simulink model "PFE_2Lignes_RNA (2)"  (R2024a)
settings: Solver=ode4  StartTime=0.0  StopTime=0.18  RelTol=1e-3
libraries: neural x202, spsRMSLib x12, spsThreePhasePISectionLineLib x4, spsThreePhaseFaultLib x2, spsThreePhaseVIMeasurementLib x2, spsThreePhaseSourceLib x2, spspowerguiLib x1
(part 6 of 10)

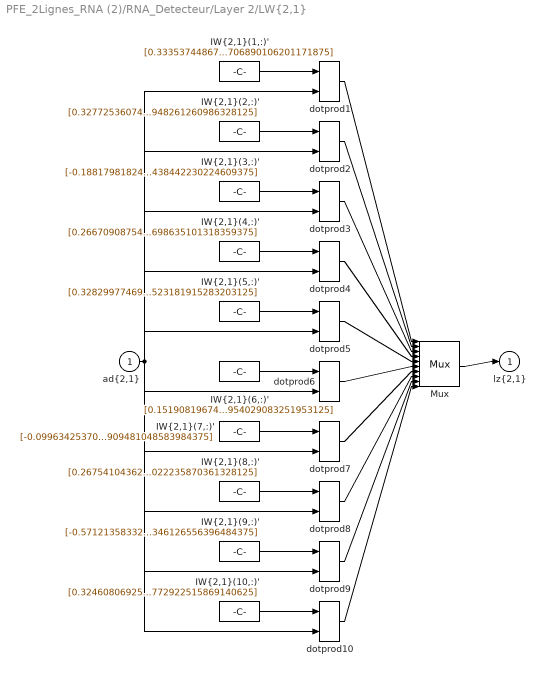
== system PFE_2Lignes_RNA (2)/RNA_Detecteur/Layer 2/LW{2,1} ==
  "ad{2,1}" : Inport  PortDimensions=20
      mask Display: e = 0.06;c1 = [120 230 180]/255;c2 = ([120 230 180]+0)/(256+128);c3 = ([120 230 180]+128)/(256+128);patch([0 1 1 0],[0 0 1 1],c1);patch([0 1 1 1-e 1-e 0+e],[0 0 1 1-e 0+e 0+e],c2);patch([0 0 1 1-e 0+e 0+e],[0 1 1 1-e 1-e 0+e],c3);plot([0 1 1 0 0],[0 0 1 1 0]);
  "IW{2,1}(1,:)'" : Constant  Value=[0.333537448675894021565824232311570085585117340087890625;0.30756652099067094408013645079336129128932952880859375;0.64409548539656069632286516934982500970363616943359375;-0.3189649752100456314707344063208438456058502197265625;0.52701815370737514765409059691592119634151458740234375;0.8021791800394260096851439811871387064456939697265625;-0.2047151820317727466402857317007146775722503662109375;0.6402572386032165940861204944667406380176544189453125;-0.38583498400512439285847676728735677897930145263671875;0.336875538549642195018662960137589834630489349365234375;-0.39560723879220571763681846277904696762561798095703125;-0.2296917297907994370831374908448196947574615478515625;-0.086281908860037670461196057658526115119457244873046875;0.75323236356745859598760262088035233318805694580078125;0.2248015108226981972894265027207438834011554718017578125;-0.50941598680687005806788647532812319695949554443359375;-0.27835551742671615915725169543293304741382598876953125;0.2520155164091217869781758054159581661224365234375;-0.04902099493881727221289423823691322468221187591552734375;-0.40351438380255089111159350068191997706890106201171875]
      mask Display: e = 0.06;c1 = [120 150 230]/255;c2 = ([120 150 230]+0)/383;c3 = ([120 150 230]+128)/383;patch([0 1 1 0],[0 0 1 1],c1);patch([0 1 1 1-e 1-e 0+e],[0 0 1 1-e 0+e 0+e],c2);patch([0 0 1 1-e 0+e 0+e],[0 1 1 1-e 1-e 0+e],c3);plot([0 1 1 0 0],[0 0 1 1 0]);disp('weights');
  "IW{2,1}(10,:)'" : Constant  Value=[0.324608069254977815720764056095504201948642730712890625;-0.2253504424986294274457776509734685532748699188232421875;-0.095126980031401797699430744614801369607448577880859375;0.51391657056152695304263033904135227203369140625;-0.421058213936082392780946292987209744751453399658203125;-0.51267445575505299348861854014103300869464874267578125;-0.443177419805164785060469512245617806911468505859375;0.54168123706777671078071989541058428585529327392578125;0.24154099575073162409211136036901734769344329833984375;0.5612737432708019280624966995674185454845428466796875;-0.1550336204058526401450279763594153337180614471435546875;-0.366469949178925336052969896627473644912242889404296875;-0.0643645953356131172995446831919252872467041015625;-0.295342281285747798591501123155467212200164794921875;0.1845011685122251166024653912245412357151508331298828125;-0.2238883823583790733113829674039152450859546661376953125;0.2272050380486201615060082303898525424301624298095703125;-0.056797317874076568011698640248141600750386714935302734375;-0.3580455383989205042638559461920522153377532958984375;-0.368046203087687262556215728181996382772922515869140625]
      mask Display: e = 0.06;c1 = [120 150 230]/255;c2 = ([120 150 230]+0)/383;c3 = ([120 150 230]+128)/383;patch([0 1 1 0],[0 0 1 1],c1);patch([0 1 1 1-e 1-e 0+e],[0 0 1 1-e 0+e 0+e],c2);patch([0 0 1 1-e 0+e 0+e],[0 1 1 1-e 1-e 0+e],c3);plot([0 1 1 0 0],[0 0 1 1 0]);disp('weights');
  "IW{2,1}(2,:)'" : Constant  Value=[0.3277253607455403727755083309602923691272735595703125;-0.303727259487383050018394214930594898760318756103515625;-0.1794389215878750831745236382630537264049053192138671875;0.1333451232571218891820308272144757211208343505859375;0.317561858062614110753685281451907940208911895751953125;-0.282004928282138578321536215298692695796489715576171875;0.50880406770246455749884262331761419773101806640625;0.451055460360104965022998158019618131220340728759765625;-0.445929464462750946296409892966039478778839111328125;-0.1048074315317428506499908280602539889514446258544921875;0.536654800038547374896324981818906962871551513671875;0.212603841472938703827111339705879800021648406982421875;0.442326673228932876202890156491775996983051300048828125;-0.1798621176049904624161257515879697166383266448974609375;-0.312184494847219717872377486855839379131793975830078125;-0.395898276604443044579539900951203890144824981689453125;0.3911142651292391914097379412851296365261077880859375;-0.4134584532279232949036895661265589296817779541015625;0.11491794031134981712849452151203877292573451995849609375;-0.462721476116461361005605112950433976948261260986328125]
      mask Display: e = 0.06;c1 = [120 150 230]/255;c2 = ([120 150 230]+0)/383;c3 = ([120 150 230]+128)/383;patch([0 1 1 0],[0 0 1 1],c1);patch([0 1 1 1-e 1-e 0+e],[0 0 1 1-e 0+e 0+e],c2);patch([0 0 1 1-e 0+e 0+e],[0 1 1 1-e 1-e 0+e],c3);plot([0 1 1 0 0],[0 0 1 1 0]);disp('weights');
  "IW{2,1}(3,:)'" : Constant  Value=[-0.188179818241801133371637888558325357735157012939453125;-0.55453958532308111895048341466463170945644378662109375;-0.06598096481666569645962994172805338166654109954833984375;0.56672277935671788728910769350477494299411773681640625;0.00817772595066590911316861678415079950354993343353271484375;0.289745744913103620010730310241342522203922271728515625;-0.74005714209394402036679139200714416801929473876953125;-0.002426520194614505653019076447662882856093347072601318359375;-0.51927162366230172896308658891939558088779449462890625;0.233250351983831649693712506632436998188495635986328125;0.189085329062525620003043513861484825611114501953125;-0.344480270084924544704563231789506971836090087890625;-0.0945918501018693513859858512660139240324497222900390625;0.417485569424939917393402311063255183398723602294921875;-0.11078253886010201723077983615439734421670436859130859375;0.036592640693072324420409557887978735379874706268310546875;0.43357957691840187663956385222263634204864501953125;-0.0515663278919384626686195360889541916549205780029296875;0.51043107861446601614119344958453439176082611083984375;0.1880911661650336019757645544814295135438442230224609375]
      mask Display: e = 0.06;c1 = [120 150 230]/255;c2 = ([120 150 230]+0)/383;c3 = ([120 150 230]+128)/383;patch([0 1 1 0],[0 0 1 1],c1);patch([0 1 1 1-e 1-e 0+e],[0 0 1 1-e 0+e 0+e],c2);patch([0 0 1 1-e 0+e 0+e],[0 1 1 1-e 1-e 0+e],c3);plot([0 1 1 0 0],[0 0 1 1 0]);disp('weights');
  "IW{2,1}(4,:)'" : Constant  Value=[0.266709087540793643444914096107822842895984649658203125;-0.443523397545111830453379297978244721889495849609375;0.0757705333284455218034736390109173953533172607421875;-0.00401999988497774018991748334883595816791057586669921875;0.1244552070836273671705640708751161582767963409423828125;0.138973141271962585818755542277358472347259521484375;0.319902609937176507504119626901228912174701690673828125;0.495518600163877998010519831950659863650798797607421875;-0.6502971852713539391288577462546527385711669921875;-0.3173570192490708929966558571322821080684661865234375;-0.226500991066371393234391007354133762419223785400390625;0.41596660078538072458087526683812029659748077392578125;0.403953739063338590487006740659126080572605133056640625;-0.296175810054605914700687208096496760845184326171875;-0.0959006738087584131857710190161014907062053680419921875;0.50529469634429380331397396730608306825160980224609375;-0.14339828104929785990151458463515155017375946044921875;0.51843118011420241675324405150604434311389923095703125;0.2380066517442346596400426506079384125769138336181640625;-0.63188259136081226241543618016294203698635101318359375]
      mask Display: e = 0.06;c1 = [120 150 230]/255;c2 = ([120 150 230]+0)/383;c3 = ([120 150 230]+128)/383;patch([0 1 1 0],[0 0 1 1],c1);patch([0 1 1 1-e 1-e 0+e],[0 0 1 1-e 0+e 0+e],c2);patch([0 0 1 1-e 0+e 0+e],[0 1 1 1-e 1-e 0+e],c3);plot([0 1 1 0 0],[0 0 1 1 0]);disp('weights');
  "IW{2,1}(5,:)'" : Constant  Value=[0.328299774696644508509280058206059038639068603515625;-0.250285615632689417697775979831931181252002716064453125;0.416213693782252425190648636998957954347133636474609375;0.368648827641874732297111449952353723347187042236328125;0.440584971244446788052329111451399512588977813720703125;0.58189913409857541015668402906158007681369781494140625;0.473473134697926900660291948952362872660160064697265625;-0.113031159270608583256034762598574161529541015625;0.284263238681224661430491096325567923486232757568359375;-0.2367412007277955032780170085970894433557987213134765625;0.468040302907570870960540787564241327345371246337890625;-0.2653546992517987757054243047605268657207489013671875;-0.2799824822428653714467827740008942782878875732421875;-0.2096327907944749713298193682931014336645603179931640625;-0.18824971855971017742348294632392935454845428466796875;-0.41792285443707977155014532399945892393589019775390625;0.143417024114028401893250475040986202657222747802734375;0.58422763334959981751381974390824325382709503173828125;0.10723926600369416972657887754394323565065860748291015625;-0.282386985463951856178965726940077729523181915283203125]
      mask Display: e = 0.06;c1 = [120 150 230]/255;c2 = ([120 150 230]+0)/383;c3 = ([120 150 230]+128)/383;patch([0 1 1 0],[0 0 1 1],c1);patch([0 1 1 1-e 1-e 0+e],[0 0 1 1-e 0+e 0+e],c2);patch([0 0 1 1-e 0+e 0+e],[0 1 1 1-e 1-e 0+e],c3);plot([0 1 1 0 0],[0 0 1 1 0]);disp('weights');
  "IW{2,1}(6,:)'" : Constant  Value=[0.1519081967420934653478781228841398842632770538330078125;0.51516544040366996082269679391174577176570892333984375;-0.1010152223416229400054788811758044175803661346435546875;-0.06244027069895498327500860114014358259737491607666015625;-0.58044306408923718176851025418727658689022064208984375;0.170936824489375249758182917503290809690952301025390625;-0.0751588627114496976577839859601226635277271270751953125;0.239715751805511245731139524650643579661846160888671875;0.08745767309729092497949665130363428033888339996337890625;-0.443244473444351638757865430306992493569850921630859375;0.1615835379780825586948367345030419528484344482421875;0.05538287547583820025209888626704923808574676513671875;0.147541059530476525996078862590366043150424957275390625;-0.471233845825062724887999365819268859922885894775390625;-0.59215372211319639017546023751492612063884735107421875;-0.06031876481770682973948538574404665268957614898681640625;-0.4666630169801633254422768004587851464748382568359375;0.1950327049742300034029796051981975324451923370361328125;0.57038392000796578340526821193634532392024993896484375;-0.58482208730008811148337599661317653954029083251953125]
      mask Display: e = 0.06;c1 = [120 150 230]/255;c2 = ([120 150 230]+0)/383;c3 = ([120 150 230]+128)/383;patch([0 1 1 0],[0 0 1 1],c1);patch([0 1 1 1-e 1-e 0+e],[0 0 1 1-e 0+e 0+e],c2);patch([0 0 1 1-e 0+e 0+e],[0 1 1 1-e 1-e 0+e],c3);plot([0 1 1 0 0],[0 0 1 1 0]);disp('weights');
  "IW{2,1}(7,:)'" : Constant  Value=[-0.09963425370726548824240609292246517725288867950439453125;0.03175940305571449406851769481363589875400066375732421875;-0.11773906029920487570361586904255091212689876556396484375;0.164361812940235108015940568293444812297821044921875;0.25709087298297250701040184139856137335300445556640625;0.615063156838253188851695085759274661540985107421875;-0.327353368077904216537632464678608812391757965087890625;-0.2154764310027114937451386822431231848895549774169921875;0.52347074933277626396233017658232711255550384521484375;-0.23928867146873089577496784841059707105159759521484375;-0.4966581007262582669881112451548688113689422607421875;-0.10163157954460259879692074491686071269214153289794921875;0.270463549589808616158137510865344665944576263427734375;0.362977153892829196291103244220721535384654998779296875;0.1568356186167213783821949846242205239832401275634765625;-0.187039700017556598243828602790017612278461456298828125;0.1005493419104231123117898505370249040424823760986328125;-0.496964309624645494967154490950633771717548370361328125;-0.65422020355979892958231403099489398300647735595703125;0.1901592060846969134413342317202477715909481048583984375]
      mask Display: e = 0.06;c1 = [120 150 230]/255;c2 = ([120 150 230]+0)/383;c3 = ([120 150 230]+128)/383;patch([0 1 1 0],[0 0 1 1],c1);patch([0 1 1 1-e 1-e 0+e],[0 0 1 1-e 0+e 0+e],c2);patch([0 0 1 1-e 0+e 0+e],[0 1 1 1-e 1-e 0+e],c3);plot([0 1 1 0 0],[0 0 1 1 0]);disp('weights');
  "IW{2,1}(8,:)'" : Constant  Value=[0.26754104362599928634836032870225608348846435546875;-0.45548887768272205978092870282125659286975860595703125;0.552668172038348171071220349404029548168182373046875;-0.498780948938208290588391946585034020245075225830078125;0.83379502578659681066852726871729828417301177978515625;-0.453799279926799303819251463210093788802623748779296875;0.405539446135224468381608176059671677649021148681640625;0.048398570299440800412948959774439572356641292572021484375;-0.0806876145479921424996661016848520375788211822509765625;-0.350725482217302986231999284427729435265064239501953125;0.2333456498075097973465830136774457059800624847412109375;0.463241498962313980047866834865999408066272735595703125;-0.477368448781201326625023284577764570713043212890625;0.325569001977186189833446405827999114990234375;0.26148951609885762170648604296729899942874908447265625;0.0118370858439038918741292860659086727537214756011962890625;-0.2353921384600821398169756548668374307453632354736328125;0.2091331848149074745801812014178722165524959564208984375;0.6396665486507284725803401670418679714202880859375;-0.038768991138495807746711108165982295759022235870361328125]
      mask Display: e = 0.06;c1 = [120 150 230]/255;c2 = ([120 150 230]+0)/383;c3 = ([120 150 230]+128)/383;patch([0 1 1 0],[0 0 1 1],c1);patch([0 1 1 1-e 1-e 0+e],[0 0 1 1-e 0+e 0+e],c2);patch([0 0 1 1-e 0+e 0+e],[0 1 1 1-e 1-e 0+e],c3);plot([0 1 1 0 0],[0 0 1 1 0]);disp('weights');
  "IW{2,1}(9,:)'" : Constant  Value=[-0.5712135833263520812153046790626831352710723876953125;-0.83067995787172732580216916176141239702701568603515625;0.32881000510872582243138140256633050739765167236328125;-0.1090741805846105749733254697275697253644466400146484375;0.51714231637292795706883907769224606454372406005859375;0.9387061813146122535300719391671009361743927001953125;0.0166470409767388825839073973611448309384286403656005859375;-0.31271667738944775027931655131396837532520294189453125;0.18835360927484134929699166605132631957530975341796875;-0.162403658322750832354586236760951578617095947265625;-0.273355462400525828225994473541504703462123870849609375;0.501369154199994060405742857255972921848297119140625;-0.805634872137981350448399098240770399570465087890625;0.391932222094814708412968684569932520389556884765625;0.0994156077144960903524406603537499904632568359375;-0.405527576371246867292796878246008418500423431396484375;0.47726248195806186824796668588533066213130950927734375;0.15084065848736383230743740568868815898895263671875;-0.46986598451183525515517658277531154453754425048828125;-0.493697886488041193242537474361597560346126556396484375]
      mask Display: e = 0.06;c1 = [120 150 230]/255;c2 = ([120 150 230]+0)/383;c3 = ([120 150 230]+128)/383;patch([0 1 1 0],[0 0 1 1],c1);patch([0 1 1 1-e 1-e 0+e],[0 0 1 1-e 0+e 0+e],c2);patch([0 0 1 1-e 0+e 0+e],[0 1 1 1-e 1-e 0+e],c3);plot([0 1 1 0 0],[0 0 1 1 0]);disp('weights');
  Mux : Mux  Inputs=10
      mask Display: e = 0.06;c1 = [120 150 230]/255;c2 = ([120 150 230]+0)/383;c3 = ([120 150 230]+128)/383;patch([0 1 1 0],[0 0 1 1],c1);patch([0 1 1 1-e 1-e 0+e],[0 0 1 1-e 0+e 0+e],c2);patch([0 0 1 1-e 0+e 0+e],[0 1 1 1-e 1-e 0+e],c3);plot([0 1 1 0 0],[0 0 1 1 0]);disp('Mux');
  dotprod{1..10} (10 alike) : neural/Weight Functions/dotprod
  "lz{2,1}" : Outport
      mask Display: e = 0.06;c1 = [120 230 180]/255;c2 = ([120 230 180]+0)/(256+128);c3 = ([120 230 180]+128)/(256+128);patch([0 1 1 0],[0 0 1 1],c1);patch([0 1 1 1-e 1-e 0+e],[0 0 1 1-e 0+e 0+e],c2);patch([0 0 1 1-e 0+e 0+e],[0 1 1 1-e 1-e 0+e],c3);plot([0 1 1 0 0],[0 0 1 1 0]);
  wires:
  "IW{2,1}(1,:)'"/1 -> dotprod1/1
  "ad{2,1}"/1 -> dotprod1/2, dotprod2/2, dotprod3/2, dotprod4/2, dotprod5/2, dotprod6/2, dotprod7/2, dotprod8/2, dotprod9/2, dotprod10/2
  dotprod1/1 -> Mux/1
  "IW{2,1}(2,:)'"/1 -> dotprod2/1
  dotprod2/1 -> Mux/2
  "IW{2,1}(3,:)'"/1 -> dotprod3/1
  dotprod3/1 -> Mux/3
  "IW{2,1}(4,:)'"/1 -> dotprod4/1
  dotprod4/1 -> Mux/4
  "IW{2,1}(5,:)'"/1 -> dotprod5/1
  dotprod5/1 -> Mux/5
  "IW{2,1}(6,:)'"/1 -> dotprod6/1
  dotprod6/1 -> Mux/6
  "IW{2,1}(7,:)'"/1 -> dotprod7/1
  dotprod7/1 -> Mux/7
  "IW{2,1}(8,:)'"/1 -> dotprod8/1
  dotprod8/1 -> Mux/8
  "IW{2,1}(9,:)'"/1 -> dotprod9/1
  dotprod9/1 -> Mux/9
  "IW{2,1}(10,:)'"/1 -> dotprod10/1
  dotprod10/1 -> Mux/10
  Mux/1 -> "lz{2,1}"/1

== system PFE_2Lignes_RNA (2)/RNA_Detecteur/Layer 3/Delays 1 ==
  "p{3}" : Inport  PortDimensions=10
      mask Display: e = 0.06;c1 = [120 230 180]/255;c2 = ([120 230 180]+0)/(256+128);c3 = ([120 230 180]+128)/(256+128);patch([0 1 1 0],[0 0 1 1],c1);patch([0 1 1 1-e 1-e 0+e],[0 0 1 1-e 0+e 0+e],c2);patch([0 0 1 1-e 0+e 0+e],[0 1 1 1-e 1-e 0+e],c3);plot([0 1 1 0 0],[0 0 1 1 0]);
  mux : Mux  Inputs=1
      mask Display: e = 0.06;c1 = [120 150 230]/255;c2 = ([120 150 230]+0)/383;c3 = ([120 150 230]+128)/383;patch([0 1 1 0],[0 0 1 1],c1);patch([0 1 1 1-e 1-e 0+e],[0 0 1 1-e 0+e 0+e],c2);patch([0 0 1 1-e 0+e 0+e],[0 1 1 1-e 1-e 0+e],c3);plot([0 1 1 0 0],[0 0 1 1 0]);disp('Mux')
  "pd{3,2}" : Outport
      mask Display: e = 0.06;c1 = [120 230 180]/255;c2 = ([120 230 180]+0)/(256+128);c3 = ([120 230 180]+128)/(256+128);patch([0 1 1 0],[0 0 1 1],c1);patch([0 1 1 1-e 1-e 0+e],[0 0 1 1-e 0+e 0+e],c2);patch([0 0 1 1-e 0+e 0+e],[0 1 1 1-e 1-e 0+e],c3);plot([0 1 1 0 0],[0 0 1 1 0]);
  wires:
  "p{3}"/1 -> mux/1
  mux/1 -> "pd{3,2}"/1

== system PFE_2Lignes_RNA (2)/RNA_Detecteur/Layer 3/LW{3,2} ==
  "ad{3,2}" : Inport  PortDimensions=10
      mask Display: e = 0.06;c1 = [120 230 180]/255;c2 = ([120 230 180]+0)/(256+128);c3 = ([120 230 180]+128)/(256+128);patch([0 1 1 0],[0 0 1 1],c1);patch([0 1 1 1-e 1-e 0+e],[0 0 1 1-e 0+e 0+e],c2);patch([0 0 1 1-e 0+e 0+e],[0 1 1 1-e 1-e 0+e],c3);plot([0 1 1 0 0],[0 0 1 1 0]);
  "IW{3,2}(1,:)'" : Constant  Value=[1.0835787994601144834660999549669213593006134033203125;0.8529235430677999385551402156124822795391082763671875;-0.2239543940285412537694043066949234344065189361572265625;0.62486299571850334455547226752969436347484588623046875;-0.2410163446748037063827041492913849651813507080078125;0.01693235877677450040845741341399843804538249969482421875;0.75220364671248052257368499340373091399669647216796875;0.9411142019242053624594745997455902397632598876953125;1.4320475692975420667352182135800831019878387451171875;-0.76515736355878483099246523124747909605503082275390625]
      mask Display: e = 0.06;c1 = [120 150 230]/255;c2 = ([120 150 230]+0)/383;c3 = ([120 150 230]+128)/383;patch([0 1 1 0],[0 0 1 1],c1);patch([0 1 1 1-e 1-e 0+e],[0 0 1 1-e 0+e 0+e],c2);patch([0 0 1 1-e 0+e 0+e],[0 1 1 1-e 1-e 0+e],c3);plot([0 1 1 0 0],[0 0 1 1 0]);disp('weights');
  "IW{3,2}(2,:)'" : Constant  Value=[-0.9088105598692874931288088191649876534938812255859375;-0.28651932989727224576625985719147138297557830810546875;-0.66772501828640873355880103190429508686065673828125;-0.63508595109610077589223919858341105282306671142578125;-0.432806848317656756019999875206849537789821624755859375;-0.312419364062227533640481169641134329140186309814453125;-0.06448079761641178908604388198000378906726837158203125;-0.286758742152342704923029259589384309947490692138671875;-0.9438796887834353110946494780364446341991424560546875;1.0782332032457004888925666818977333605289459228515625]
      mask Display: e = 0.06;c1 = [120 150 230]/255;c2 = ([120 150 230]+0)/383;c3 = ([120 150 230]+128)/383;patch([0 1 1 0],[0 0 1 1],c1);patch([0 1 1 1-e 1-e 0+e],[0 0 1 1-e 0+e 0+e],c2);patch([0 0 1 1-e 0+e 0+e],[0 1 1 1-e 1-e 0+e],c3);plot([0 1 1 0 0],[0 0 1 1 0]);disp('weights');
  Mux : Mux  Inputs=2
      mask Display: e = 0.06;c1 = [120 150 230]/255;c2 = ([120 150 230]+0)/383;c3 = ([120 150 230]+128)/383;patch([0 1 1 0],[0 0 1 1],c1);patch([0 1 1 1-e 1-e 0+e],[0 0 1 1-e 0+e 0+e],c2);patch([0 0 1 1-e 0+e 0+e],[0 1 1 1-e 1-e 0+e],c3);plot([0 1 1 0 0],[0 0 1 1 0]);disp('Mux');
  dotprod1 : neural/Weight Functions/dotprod
  dotprod2 : neural/Weight Functions/dotprod
  "lz{3,2}" : Outport
      mask Display: e = 0.06;c1 = [120 230 180]/255;c2 = ([120 230 180]+0)/(256+128);c3 = ([120 230 180]+128)/(256+128);patch([0 1 1 0],[0 0 1 1],c1);patch([0 1 1 1-e 1-e 0+e],[0 0 1 1-e 0+e 0+e],c2);patch([0 0 1 1-e 0+e 0+e],[0 1 1 1-e 1-e 0+e],c3);plot([0 1 1 0 0],[0 0 1 1 0]);
  wires:
  "IW{3,2}(1,:)'"/1 -> dotprod1/1
  "ad{3,2}"/1 -> dotprod1/2, dotprod2/2
  dotprod1/1 -> Mux/1
  "IW{3,2}(2,:)'"/1 -> dotprod2/1
  dotprod2/1 -> Mux/2
  Mux/1 -> "lz{3,2}"/1

== system PFE_2Lignes_RNA (2)/RNA_Localisateur/Layer 1/Delays 1 ==
  "p{1}" : Inport  PortDimensions=12
      mask Display: e = 0.06;c1 = [120 230 180]/255;c2 = ([120 230 180]+0)/(256+128);c3 = ([120 230 180]+128)/(256+128);patch([0 1 1 0],[0 0 1 1],c1);patch([0 1 1 1-e 1-e 0+e],[0 0 1 1-e 0+e 0+e],c2);patch([0 0 1 1-e 0+e 0+e],[0 1 1 1-e 1-e 0+e],c3);plot([0 1 1 0 0],[0 0 1 1 0]);
  mux : Mux  Inputs=1
      mask Display: e = 0.06;c1 = [120 150 230]/255;c2 = ([120 150 230]+0)/383;c3 = ([120 150 230]+128)/383;patch([0 1 1 0],[0 0 1 1],c1);patch([0 1 1 1-e 1-e 0+e],[0 0 1 1-e 0+e 0+e],c2);patch([0 0 1 1-e 0+e 0+e],[0 1 1 1-e 1-e 0+e],c3);plot([0 1 1 0 0],[0 0 1 1 0]);disp('Mux')
  "pd{1,1}" : Outport
      mask Display: e = 0.06;c1 = [120 230 180]/255;c2 = ([120 230 180]+0)/(256+128);c3 = ([120 230 180]+128)/(256+128);patch([0 1 1 0],[0 0 1 1],c1);patch([0 1 1 1-e 1-e 0+e],[0 0 1 1-e 0+e 0+e],c2);patch([0 0 1 1-e 0+e 0+e],[0 1 1 1-e 1-e 0+e],c3);plot([0 1 1 0 0],[0 0 1 1 0]);
  wires:
  "p{1}"/1 -> mux/1
  mux/1 -> "pd{1,1}"/1
